simulink model "CT_EOPLL"  (R2021b)
settings: Solver=FixedStepAuto  StartTime=0.0  StopTime=1e-2  FixedStep=1e-11  RelTol=1e-3
values from neighbouring files (symbols this model uses):
  f0 = 5e9    (= 5000000000)    [CT_EOPLL.m]    (also in DT_EOPLL.m = 50000000000)
  h0 = 1e4    (= 10000)    [CT_EOPLL.m]    (also in DT_EOPLL.m)
  K_int = 10    [CT_EOPLL.m]    (also in DT_EOPLL.m)
  K_loop = 3.33e-3    (= 0.00333)    [CT_EOPLL.m]    (also in DT_EOPLL.m = 10)
  Kf = 1e13    (= 10000000000000)    [CT_EOPLL.m]    (also in DT_EOPLL.m)
  p0 = 1    [CT_EOPLL.m]    (also in DT_EOPLL.m)
  R = 1    [CT_EOPLL.m]    (also in DT_EOPLL.m)
  T_meas = 2e-4    (= 0.0002)    [CT_EOPLL.m]    (also in DT_EOPLL.m)
  t_mzi = 2e-9    (= 2e-09)    [CT_EOPLL.m]    (also in DT_EOPLL.m = 2e-08)
  w_int = 2*pi*300    (= 1884.95559215)    [CT_EOPLL.m]    (also in DT_EOPLL.m)
  w_ref = 2*pi*2e5    (= 1256637.06144)    [CT_EOPLL.m]
  wf = 2*pi*1e7    (= 62831853.0718)    [CT_EOPLL.m]    (also in DT_EOPLL.m)
undefined symbols (not defined in the file or in its folder): K_coupler, magnitude
libraries: phaseddetectlib x2, simulink x1
settings Model: Creator=Marziyeh Rezaei  LastModifiedBy=Marziyeh Rezaei

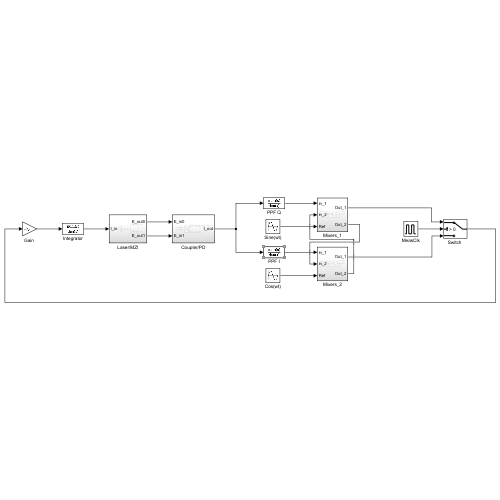
[thumbnail: Simulink's stored preview of the top-level diagram]
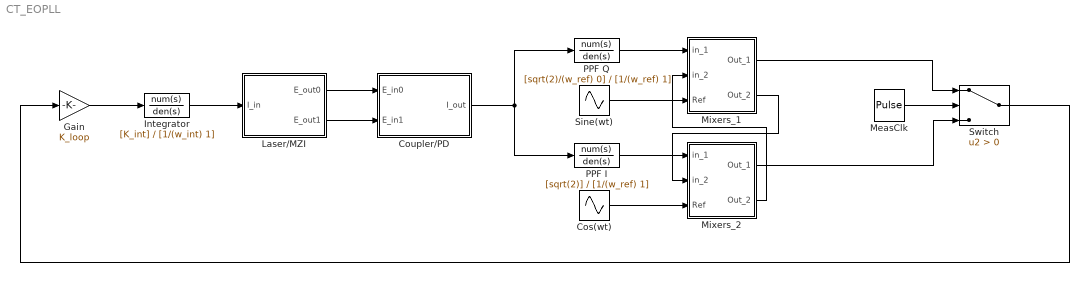
== system CT_EOPLL ==
  Cos(wt) : Sin  Frequency=w_ref  Phase=pi/2  SampleTime=0
  Coupler/PD : Subsystem
  "Gain " : Gain  Gain=K_loop
  Integrator : TransferFcn  Numerator=[K_int]  Denominator=[1/(w_int) 1]
  Laser/MZI : Subsystem
  MeasClk : DiscretePulseGenerator  PulseType=Time based  Period=T_meas  PulseWidth=50
  Mixers_1 : Subsystem
  Mixers_2 : Subsystem
  PPF I : TransferFcn  Numerator=[sqrt(2)]  Denominator=[1/(w_ref) 1]
  PPF Q : TransferFcn  Numerator=[sqrt(2)/(w_ref) 0]  Denominator=[1/(w_ref) 1]
  Sine(wt) : Sin  Frequency=w_ref  SampleTime=0
  "Switch " : Switch  Criteria=u2 > Threshold
  wires:
  "Switch "/1 -> "Gain "/1
  MeasClk/1 -> "Switch "/2
  "Gain "/1 -> Integrator/1
  PPF I/1 -> Mixers_2/1(in_1)
  Mixers_1/2(Out_2) -> Mixers_2/2(in_2)
  Mixers_2/1(Out_1) -> "Switch "/3
  Mixers_2/2(Out_2) -> Mixers_1/2(in_2)
  PPF Q/1 -> Mixers_1/1(in_1)
  Mixers_1/1(Out_1) -> "Switch "/1
  Coupler/PD/1(I_out) -> PPF I/1, PPF Q/1
  Integrator/1 -> Laser/MZI/1(I_in)
  Laser/MZI/1(E_out0) -> Coupler/PD/1(E_in0)
  Laser/MZI/2(E_out1) -> Coupler/PD/2(E_in1)
  Sine(wt)/1 -> Mixers_1/3(Ref)
  Cos(wt)/1 -> Mixers_2/3(Ref)

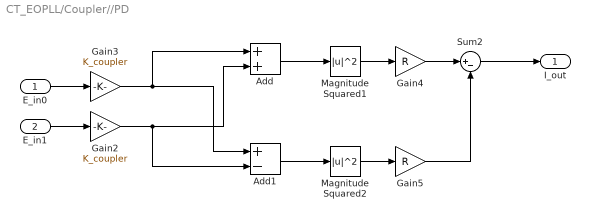
== system CT_EOPLL/Coupler//PD ==
  E_in0 : Inport
  E_in1 : Inport  Port=2
  Add : Sum
  Add1 : Sum  Inputs=+-
  Gain2 : Gain  Gain=K_coupler
  Gain3 : Gain  Gain=K_coupler
  Gain4 : Gain  Gain=R
  Gain5 : Gain  Gain=R
  Magnitude Squared1 : Math  Operator=magnitude^2  SaturateOnIntegerOverflow=on
  Magnitude Squared2 : Math  Operator=magnitude^2  SaturateOnIntegerOverflow=on
  Sum2 : Sum  Inputs=|+-
  I_out : Outport
  wires:
  Add1/1 -> Magnitude Squared2/1
  Add/1 -> Magnitude Squared1/1
  E_in1/1 -> Gain2/1
  Magnitude Squared1/1 -> Gain4/1
  Gain5/1 -> Sum2/2
  E_in0/1 -> Gain3/1
  Magnitude Squared2/1 -> Gain5/1
  Gain2/1 -> Add/2, Add1/2
  Gain4/1 -> Sum2/1
  Gain3/1 -> Add1/1, Add/1
  Sum2/1 -> I_out/1

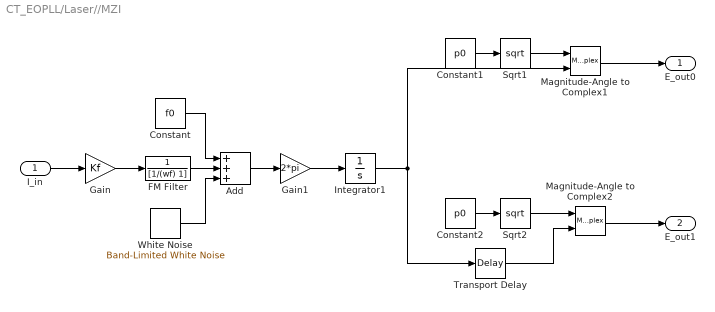
== system CT_EOPLL/Laser//MZI ==
  I_in : Inport
  Add : Sum  Inputs=+++
  Constant : Constant  Value=f0
  Constant1 : Constant  Value=p0
  Constant2 : Constant  Value=p0
  FM Filter : TransferFcn  Denominator=[1/(wf) 1]
  Gain : Gain  Gain=Kf
  Gain1 : Gain  Gain=2*pi
  Integrator1 : Integrator
  Magnitude-Angle to Complex1 : MagnitudeAngleToComplex
  Magnitude-Angle to Complex2 : MagnitudeAngleToComplex
  Sqrt1 : Sqrt  SaturateOnIntegerOverflow=on
  Sqrt2 : Sqrt  SaturateOnIntegerOverflow=on
  Transport Delay : TransportDelay  DelayTime=t_mzi
  White Noise : simulink/Sources/Band-Limited White Noise  Cov=[h0]  Ts=1e-7  seed=[23341]
  E_out0 : Outport
  E_out1 : Outport  Port=2
  wires:
  Gain1/1 -> Integrator1/1
  Sqrt2/1 -> Magnitude-Angle to Complex2/1
  Sqrt1/1 -> Magnitude-Angle to Complex1/1
  Constant2/1 -> Sqrt2/1
  Magnitude-Angle to Complex1/1 -> E_out0/1
  Magnitude-Angle to Complex2/1 -> E_out1/1
  Constant1/1 -> Sqrt1/1
  I_in/1 -> Gain/1
  Gain/1 -> FM Filter/1
  Transport Delay/1 -> Magnitude-Angle to Complex2/2
  Integrator1/1 -> Magnitude-Angle to Complex1/2, Transport Delay/1
  Add/1 -> Gain1/1
  FM Filter/1 -> Add/2
  Constant/1 -> Add/1
  White Noise/1 -> Add/3

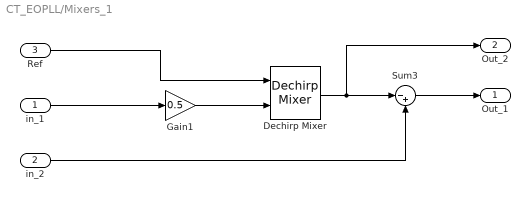
== system CT_EOPLL/Mixers_1 ==
  in_1 : Inport
  in_2 : Inport  Port=2
  Ref : Inport  Port=3
  Dechirp Mixer : phaseddetectlib/Dechirp Mixer
      settings: SourceProductBaseCode=AR
  Gain1 : Gain  Gain=0.5
  Sum3 : Sum  Inputs=|-+
  Out_1 : Outport
  Out_2 : Outport  Port=2
  wires:
  Gain1/1 -> Dechirp Mixer/2
  Ref/1 -> Dechirp Mixer/1
  in_1/1 -> Gain1/1
  Sum3/1 -> Out_1/1
  in_2/1 -> Sum3/2
  Dechirp Mixer/1 -> Out_2/1, Sum3/1

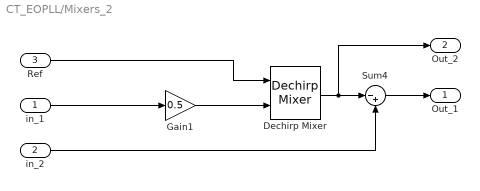
== system CT_EOPLL/Mixers_2 ==
  in_1 : Inport
  in_2 : Inport  Port=2
  Ref : Inport  Port=3
  Dechirp Mixer : phaseddetectlib/Dechirp Mixer
      settings: SourceProductBaseCode=AR
  Gain1 : Gain  Gain=0.5
  Sum4 : Sum  Inputs=|-+
  Out_1 : Outport
  Out_2 : Outport  Port=2
  wires:
  Gain1/1 -> Dechirp Mixer/2
  Ref/1 -> Dechirp Mixer/1
  in_1/1 -> Gain1/1
  Sum4/1 -> Out_1/1
  in_2/1 -> Sum4/2
  Dechirp Mixer/1 -> Out_2/1, Sum4/1
